simulink library "Energy_converter_Electrical_to_Mechanical"  (R2016a)
settings: Solver=ode1  StartTime=0.0  StopTime=Inf  FixedStep=0.001  RelTol=1e-3
undefined symbols (not defined in the file): API1dcac_efficiency, API2dcac_efficiency, API3dcac_efficiency, aux_power_state, AWR_InvStError, dat, DiscIntNeverNeededParam, EDCU_p_RefTqeMOT, emot_AcCmprFront_inertia, emot_AcCmprFront_nTab_3rdD, emot_AcCmprFront_pwrAC, emot_AcCmprFront_Tau, emot_AcCmprFront_trqTab_2ndD, emot_AcCmprFront_vltTab_1stD, emot_AcCmprRear_inertia, emot_AcCmprRear_nTab_3rdD, emot_AcCmprRear_pwrAC, emot_AcCmprRear_Tau, emot_AcCmprRear_trqTab_2ndD, emot_AcCmprRear_vltTab_1stD, emot_AirCmpr_inertia, emot_AirCmpr_nTab_3rdD, emot_AirCmpr_pwrAC, emot_AirCmpr_Tau, emot_AirCmpr_trqTab_2ndD, emot_AirCmpr_vltTab_1stD, emot_aircomp_power, emot_Cth_rotor, emot_Cth_stator, emot_dtrqEmotNeg, emot_dtrqEmotPtv, emot_inv_pwracTab_1st, emot_inv_pwrDC, emot_inv_pwrLoss, emot_inv_VrmsTab_2nd, emot_j, emot_mot_pwrLoss, emot_nTab_1stD, emot_pwrEtaTab_nRow, emot_pwrEtaTab_pwrTab, emot_pwrEtaTab_trqClm, emot_Rth_rotor_oil, emot_Rth_stator_oil, emot_Rth_stator_rotor, emot_tractiongroup, emot_Trotor_init, emot_trqMaxRow, emot_trqMinRow, emot_Tstator_init, emot_vltTab_3rdD, FirstDrivenAxleNoOfEmot, inv_Cth_cooling_plate, inv_Cth_diode, inv_Cth_IGBT, inv_n_IGBT_per_Switch, inv_Rth_cooling_plate_coolant, inv_Rth_PS_cooling_plate, inv_Tplate_init, inv_Tpowerstack_init, midAxleNoOfEmot ... (+6)
libraries: Electrical_converter x12, Energy_converter_Electrical_to_Mechanical x12, simulink x7
(part 4 of 8)

== system Energy_converter_Electrical_to_Mechanical/AWR_DriveEmot/EMD1_CMD_Command2 ==
  EMD1_CMD_ClearErrors : Inport
  EMD1_CMD_MotorControlMode : Inport  Port=2
  Compare To Constant : Subsystem  mask(Compare To Constant){relop===, const=1, OutDataTypeStr=boolean, ZeroCross=on}
      mask prompts: relop "Simulink:masks:Operator_MP"; const "Simulink:masks:ConstantValue_MP"; OutDataTypeStr "Simulink:masks:OutputDataType_MP"; ZeroCross "Simulink:masks:EnableZerocrossingDetection_MP"
      mask help: Simulink:masks:CompareToConstant_MD
      mask init: same as Energy_converter_Electrical_to_Mechanical/AWR_DriveEmot/EMD1_CMD_Command/Compare To Constant
      mask TypeOptions relop: == | ~= | < | <= | >= | >
      mask TypeOptions OutDataTypeStr: Simulink:masks:uint8 | Simulink:masks:boolean
      mask Callback ZeroCross: sl('zeroCrossEnable', gcbh);
      mask Display: disp(str)
  Compare To Constant1 : Subsystem  mask(Compare To Constant){relop===, const=1, OutDataTypeStr=boolean, ZeroCross=on}
      mask prompts: relop "Simulink:masks:Operator_MP"; const "Simulink:masks:ConstantValue_MP"; OutDataTypeStr "Simulink:masks:OutputDataType_MP"; ZeroCross "Simulink:masks:EnableZerocrossingDetection_MP"
      mask help: Simulink:masks:CompareToConstant_MD
      mask init: same as Energy_converter_Electrical_to_Mechanical/AWR_DriveEmot/EMD1_CMD_Command/Compare To Constant
      mask TypeOptions relop: == | ~= | < | <= | >= | >
      mask TypeOptions OutDataTypeStr: Simulink:masks:uint8 | Simulink:masks:boolean
      mask Callback ZeroCross: sl('zeroCrossEnable', gcbh);
      mask Display: disp(str)
  Constant : Constant  Value=4
  Constant3 : Constant
  Constant4 : Constant  Value=0
  Switch : Switch  Threshold=0.5
  Switch1 : Switch  Threshold=0.5
  Out_EMD1_CMD_Command : Outport
  wires:
  EMD1_CMD_MotorControlMode/1 -> Compare To Constant/1(u)
  EMD1_CMD_ClearErrors/1 -> Compare To Constant1/1(u)
  Compare To Constant1/1(y) -> Switch/2
  Switch1/1 -> Switch/3
  Constant/1 -> Switch/1
  Constant3/1 -> Switch1/1
  Constant4/1 -> Switch1/3
  Switch/1 -> Out_EMD1_CMD_Command/1
  Compare To Constant/1(y) -> Switch1/2

== system Energy_converter_Electrical_to_Mechanical/AWR_DriveEmot/EMD1_CMD_Command3 ==
  EMD1_CMD_ClearErrors : Inport
  EMD1_CMD_MotorControlMode : Inport  Port=2
  Compare To Constant : Subsystem  mask(Compare To Constant){relop===, const=1, OutDataTypeStr=boolean, ZeroCross=on}
      mask prompts: relop "Simulink:masks:Operator_MP"; const "Simulink:masks:ConstantValue_MP"; OutDataTypeStr "Simulink:masks:OutputDataType_MP"; ZeroCross "Simulink:masks:EnableZerocrossingDetection_MP"
      mask help: Simulink:masks:CompareToConstant_MD
      mask init: same as Energy_converter_Electrical_to_Mechanical/AWR_DriveEmot/EMD1_CMD_Command/Compare To Constant
      mask TypeOptions relop: == | ~= | < | <= | >= | >
      mask TypeOptions OutDataTypeStr: Simulink:masks:uint8 | Simulink:masks:boolean
      mask Callback ZeroCross: sl('zeroCrossEnable', gcbh);
      mask Display: disp(str)
  Compare To Constant1 : Subsystem  mask(Compare To Constant){relop===, const=1, OutDataTypeStr=boolean, ZeroCross=on}
      mask prompts: relop "Simulink:masks:Operator_MP"; const "Simulink:masks:ConstantValue_MP"; OutDataTypeStr "Simulink:masks:OutputDataType_MP"; ZeroCross "Simulink:masks:EnableZerocrossingDetection_MP"
      mask help: Simulink:masks:CompareToConstant_MD
      mask init: same as Energy_converter_Electrical_to_Mechanical/AWR_DriveEmot/EMD1_CMD_Command/Compare To Constant
      mask TypeOptions relop: == | ~= | < | <= | >= | >
      mask TypeOptions OutDataTypeStr: Simulink:masks:uint8 | Simulink:masks:boolean
      mask Callback ZeroCross: sl('zeroCrossEnable', gcbh);
      mask Display: disp(str)
  Constant : Constant  Value=4
  Constant3 : Constant
  Constant4 : Constant  Value=0
  Switch : Switch  Threshold=0.5
  Switch1 : Switch  Threshold=0.5
  Out_EMD1_CMD_Command : Outport
  wires:
  EMD1_CMD_MotorControlMode/1 -> Compare To Constant/1(u)
  EMD1_CMD_ClearErrors/1 -> Compare To Constant1/1(u)
  Compare To Constant1/1(y) -> Switch/2
  Switch1/1 -> Switch/3
  Constant/1 -> Switch/1
  Constant3/1 -> Switch1/1
  Constant4/1 -> Switch1/3
  Switch/1 -> Out_EMD1_CMD_Command/1
  Compare To Constant/1(y) -> Switch1/2

== system Energy_converter_Electrical_to_Mechanical/AWR_DriveEmot/Emot1_4 ==
  hvs_emot_Emot1_angVel : Inport
  voltBatHV1 : Inport  Port=2
  trqEmotDesPhy1 : Inport  Port=3
  emot_CMD1 : Inport  Port=4
  voltBatHV4 : Inport  Port=5
  trqEmotDesPhy4 : Inport  Port=6
  emot_CMD4 : Inport  Port=7
  hvs_drvEmot1Oil_Temperature : Inport  Port=8
  inv_coolant_temperature : Inport  Port=9
  Emot1_Selection : Inport  Port=10
  Emot4_Selection : Inport  Port=11
  hvs_emot_Emot4_angVel : Inport  Port=12
  hvs_drvEmot4Oil_Temperature : Inport  Port=13
  Bus Creator1 : BusCreator  Inputs=9
  Bus Creator2 : BusCreator  Inputs=9
  Bus Creator3 : BusCreator  Inputs=2
  e-Motor1 : Energy_converter_Electrical_to_Mechanical/e-Motor  SystemSampleTime=-1
  e-Motor4 : Energy_converter_Electrical_to_Mechanical/e-Motor  SystemSampleTime=-1
  emot1_4B : Outport
  wires:
  hvs_drvEmot4Oil_Temperature/1 -> e-Motor4/5
  Emot1_Selection/1 -> e-Motor1/Enable
  Emot4_Selection/1 -> e-Motor4/Enable
  Bus Creator3/1 -> emot1_4B/1  "emot1_4B"
  trqEmotDesPhy4/1 -> e-Motor4/3
  Bus Creator2/1 -> Bus Creator3/2  "emot4B"
  Bus Creator1/1 -> Bus Creator3/1  "emot1B"
  voltBatHV4/1 -> e-Motor4/2
  hvs_emot_Emot4_angVel/1 -> e-Motor4/1
  voltBatHV1/1 -> e-Motor1/2
  trqEmotDesPhy1/1 -> e-Motor1/3
  hvs_emot_Emot1_angVel/1 -> e-Motor1/1
  e-Motor1/3 -> Bus Creator1/3
  e-Motor1/4 -> Bus Creator1/4
  e-Motor1/1 -> Bus Creator1/1
  e-Motor1/2 -> Bus Creator1/2
  e-Motor1/5 -> Bus Creator1/5
  e-Motor4/1 -> Bus Creator2/1
  e-Motor4/2 -> Bus Creator2/2
  e-Motor4/3 -> Bus Creator2/3
  e-Motor4/4 -> Bus Creator2/4
  e-Motor4/5 -> Bus Creator2/5
  emot_CMD1/1 -> e-Motor1/4
  emot_CMD4/1 -> e-Motor4/4
  inv_coolant_temperature/1 -> e-Motor1/6, e-Motor4/6
  hvs_drvEmot1Oil_Temperature/1 -> e-Motor1/5
  e-Motor1/6 -> Bus Creator1/6
  e-Motor1/7 -> Bus Creator1/7
  e-Motor1/9 -> Bus Creator1/9
  e-Motor1/8 -> Bus Creator1/8
  e-Motor4/6 -> Bus Creator2/6
  e-Motor4/7 -> Bus Creator2/7
  e-Motor4/8 -> Bus Creator2/8
  e-Motor4/9 -> Bus Creator2/9

== system Energy_converter_Electrical_to_Mechanical/AWR_DriveEmot/Emot2_3 ==
  hvs_emot_Emot2_angVel : Inport
  voltBatHV2 : Inport  Port=2
  trqEmotDesPhy2 : Inport  Port=3
  emot_CMD2 : Inport  Port=4
  voltBatHV3 : Inport  Port=5
  trqEmotDesPhy3 : Inport  Port=6
  emot_CMD3 : Inport  Port=7
  hvs_drvEmot2Oil_Temperature : Inport  Port=8
  inv_coolant_temperature : Inport  Port=9
  Emot2_Selection : Inport  Port=10
  Emot3_Selection : Inport  Port=11
  hvs_emot_Emot3_angVel : Inport  Port=12
  hvs_drvEmot3Oil_Temperature : Inport  Port=13
  Bus Creator1 : BusCreator  Inputs=9
  Bus Creator2 : BusCreator  Inputs=9
  Bus Creator3 : BusCreator  Inputs=2
  e-Motor2 : Energy_converter_Electrical_to_Mechanical/e-Motor  SystemSampleTime=-1
  e-Motor3 : Energy_converter_Electrical_to_Mechanical/e-Motor  SystemSampleTime=-1
  emot2_3B : Outport
  wires:
  hvs_drvEmot3Oil_Temperature/1 -> e-Motor3/5
  Emot3_Selection/1 -> e-Motor3/Enable
  Emot2_Selection/1 -> e-Motor2/Enable
  emot_CMD3/1 -> e-Motor3/4
  emot_CMD2/1 -> e-Motor2/4
  e-Motor3/5 -> Bus Creator2/5
  e-Motor3/4 -> Bus Creator2/4
  e-Motor3/3 -> Bus Creator2/3
  e-Motor3/2 -> Bus Creator2/2
  e-Motor3/1 -> Bus Creator2/1
  e-Motor2/5 -> Bus Creator1/5
  e-Motor2/2 -> Bus Creator1/2
  e-Motor2/1 -> Bus Creator1/1
  e-Motor2/4 -> Bus Creator1/4
  e-Motor2/3 -> Bus Creator1/3
  hvs_emot_Emot2_angVel/1 -> e-Motor2/1
  trqEmotDesPhy2/1 -> e-Motor2/3
  voltBatHV2/1 -> e-Motor2/2
  hvs_emot_Emot3_angVel/1 -> e-Motor3/1
  voltBatHV3/1 -> e-Motor3/2
  Bus Creator1/1 -> Bus Creator3/1  "emot2B"
  Bus Creator2/1 -> Bus Creator3/2  "emot3B"
  trqEmotDesPhy3/1 -> e-Motor3/3
  Bus Creator3/1 -> emot2_3B/1  "emot2_3B"
  hvs_drvEmot2Oil_Temperature/1 -> e-Motor2/5
  inv_coolant_temperature/1 -> e-Motor2/6, e-Motor3/6
  e-Motor3/7 -> Bus Creator2/7
  e-Motor3/6 -> Bus Creator2/6
  e-Motor3/8 -> Bus Creator2/8
  e-Motor3/9 -> Bus Creator2/9
  e-Motor2/6 -> Bus Creator1/6
  e-Motor2/7 -> Bus Creator1/7
  e-Motor2/9 -> Bus Creator1/9
  e-Motor2/8 -> Bus Creator1/8

== system Energy_converter_Electrical_to_Mechanical/AWR_DriveEmot/MotorSelection ==
  MidAxle : Constant  Value=FirstDrivenAxleNoOfEmot
  RearAxle : Constant  Value=SecondDrivenAxleNoOfEmot
  Truth Table : Truth Table  TreatAsAtomicUnit=on
  Emot1_Selection : Outport
  Emot2_Selection : Outport  Port=2
  Emot3_Selection : Outport  Port=3
  Emot4_Selection : Outport  Port=4
  wires:
  Truth Table/4(y4) -> Emot4_Selection/1
  Truth Table/3(y3) -> Emot3_Selection/1
  Truth Table/2(y2) -> Emot2_Selection/1
  Truth Table/1(y1) -> Emot1_Selection/1
  RearAxle/1 -> Truth Table/2(u2)
  MidAxle/1 -> Truth Table/1(u1)

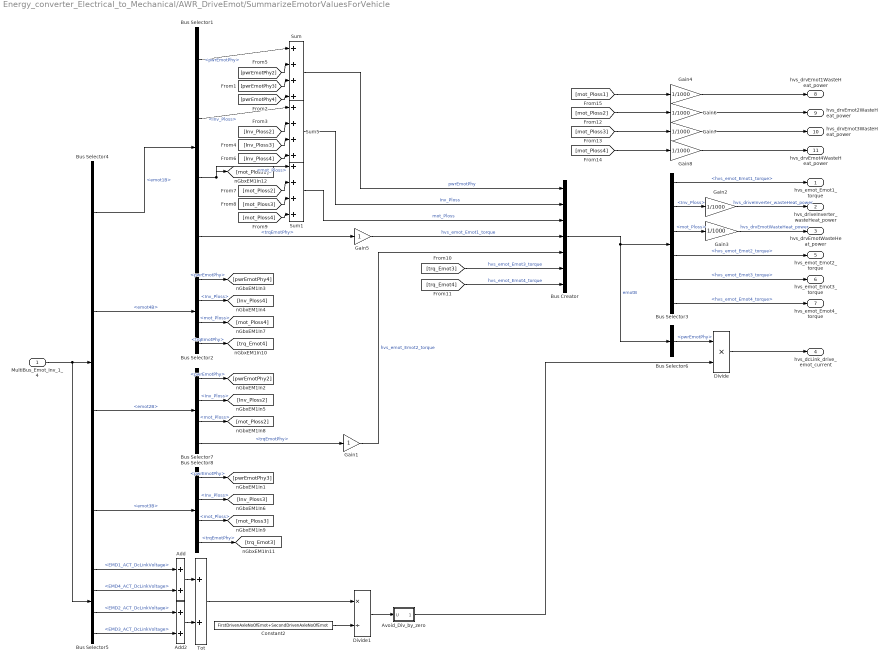
== system Energy_converter_Electrical_to_Mechanical/AWR_DriveEmot/SummarizeEmotorValuesForVehicle ==
  MultiBus_Emot_Inv_1_4 : Inport
  Add : Sum
  Add2 : Sum
  Avoid_Div_by_zero : Subsystem
  Bus Creator : BusCreator  Inputs=7
  Bus Selector{1..2,7..8} (4 alike) : BusSelector  OutputSignals=pwrEmotPhy,Inv_Ploss,mot_Ploss,trqEmotPhy
  Bus Selector3 : BusSelector  OutputSignals=hvs_emot_Emot1_torque,Inv_Ploss,mot_Ploss,hvs_emot_Emot2_torque,hvs_emot_Emot3_torque,hvs_emot_Emot4_torque
  Bus Selector4 : BusSelector  OutputSignals=emot1_4B.emot1B,emot1_4B.emot4B,emot2_3B.emot2B,emot2_3B.emot3B
  Bus Selector5 : BusSelector  OutputSignals=awr1_4B.awr1B.EMD1_ACT_DcLinkVoltage,awr1_4B.awr4B.EMD4_ACT_DcLinkVoltage,awr2_3B.awr2B.EMD2_ACT_DcLinkVoltage,awr2_3B.awr3B.EMD3_ACT_DcLinkVoltage
  Bus Selector6 : BusSelector  OutputSignals=pwrEmotPhy
  Constant2 : Constant  Value=FirstDrivenAxleNoOfEmot+SecondDrivenAxleNoOfEmot
  Divide : Product  Inputs=**
  Divide1 : Product  Inputs=*/
  Gain1 : Gain
  Gain{2..4,6..8} (6 alike) : Gain  Gain=1/1000
  Gain5 : Gain
  Sum : Sum  Inputs=|++++
  Sum1 : Sum  Inputs=|++++
  Sum5 : Sum  Inputs=|++++
  Tot : Sum
  hvs_emot_Emot1_torque : Outport
  hvs_driveInverter_wasteHeat_power : Outport  Port=2
  hvs_drvEmotWasteHeat_power : Outport  Port=3
  hvs_dcLink_drive_emot_current : Outport  Port=4
  hvs_emot_Emot2_torque : Outport  Port=5
  hvs_emot_Emot3_torque : Outport  Port=6
  hvs_emot_Emot4_torque : Outport  Port=7
  hvs_drvEmot1WasteHeat_power : Outport  Port=8
  hvs_drvEmot2WasteHeat_power : Outport  Port=9
  hvs_drvEmot3WasteHeat_power : Outport  Port=10
  hvs_drvEmot4WasteHeat_power : Outport  Port=11
  wires:
  Gain8/1 -> hvs_drvEmot4WasteHeat_power/1
  Gain7/1 -> hvs_drvEmot3WasteHeat_power/1
  Gain6/1 -> hvs_drvEmot2WasteHeat_power/1
  Gain4/1 -> hvs_drvEmot1WasteHeat_power/1
  [mot_Ploss4] -> Gain8/1
  [mot_Ploss3] -> Gain7/1
  [mot_Ploss2] -> Gain6/1
  [mot_Ploss1] -> Gain4/1
  Bus Selector3/6 -> hvs_emot_Emot4_torque/1  "<hvs_emot_Emot4_torque>"
  Bus Selector3/5 -> hvs_emot_Emot3_torque/1  "<hvs_emot_Emot3_torque>"
  Bus Selector3/4 -> hvs_emot_Emot2_torque/1  "<hvs_emot_Emot2_torque>"
  Bus Selector3/1 -> hvs_emot_Emot1_torque/1  "<hvs_emot_Emot1_torque>"
  [trq_Emot4] -> Bus Creator/7  "hvs_emot_Emot4_torque"
  [trq_Emot3] -> Bus Creator/6  "hvs_emot_Emot3_torque"
  Bus Selector2/4 -> [trq_Emot4]  "<trqEmotPhy>"
  Tot/1 -> Divide1/1
  Constant2/1 -> Divide1/2
  Add2/1 -> Tot/2
  Bus Selector5/4 -> Add2/2  "<EMD3_ACT_DcLinkVoltage>"
  Bus Selector5/3 -> Add2/1  "<EMD2_ACT_DcLinkVoltage>"
  Gain1/1 -> Bus Creator/5  "hvs_emot_Emot2_torque"
  Bus Selector8/4 -> [trq_Emot3]  "<trqEmotPhy>"
  Bus Selector7/4 -> Gain1/1  "<trqEmotPhy>"
  [mot_Ploss4] -> Sum1/4
  [mot_Ploss3] -> Sum1/3
  [mot_Ploss2] -> Sum1/2
  Bus Selector8/3 -> [mot_Ploss3]  "<mot_Ploss>"
  Bus Selector7/3 -> [mot_Ploss2]  "<mot_Ploss>"
  Bus Selector8/2 -> [Inv_Ploss3]  "<Inv_Ploss>"
  Bus Selector7/2 -> [Inv_Ploss2]  "<Inv_Ploss>"
  [Inv_Ploss4] -> Sum5/4
  [Inv_Ploss3] -> Sum5/3
  [Inv_Ploss2] -> Sum5/2
  [pwrEmotPhy4] -> Sum/4
  [pwrEmotPhy3] -> Sum/3
  [pwrEmotPhy2] -> Sum/2
  Bus Selector2/1 -> [pwrEmotPhy4]  "<pwrEmotPhy>"
  Bus Selector8/1 -> [pwrEmotPhy3]  "<pwrEmotPhy>"
  Bus Selector7/1 -> [pwrEmotPhy2]  "<pwrEmotPhy>"
  Bus Selector4/3 -> Bus Selector7/1  "<emot2B>"
  Bus Selector4/4 -> Bus Selector8/1  "<emot3B>"
  Gain3/1 -> hvs_drvEmotWasteHeat_power/1  "hvs_drvEmotWasteHeat_power"
  Bus Selector3/3 -> Gain3/1  "<mot_Ploss>"
  Gain2/1 -> hvs_driveInverter_wasteHeat_power/1  "hvs_driveInverter_wasteHeat_power"
  Bus Selector3/2 -> Gain2/1  "<Inv_Ploss>"
  Divide/1 -> hvs_dcLink_drive_emot_current/1
  Avoid_Div_by_zero/1(1/U) -> Divide/2
  Bus Selector6/1 -> Divide/1  "<pwrEmotPhy>"
  Divide1/1 -> Avoid_Div_by_zero/1(U)
  Add/1 -> Tot/1
  Bus Selector5/2 -> Add/2  "<EMD4_ACT_DcLinkVoltage>"
  Bus Selector5/1 -> Add/1  "<EMD1_ACT_DcLinkVoltage>"
  Bus Creator/1 -> Bus Selector6/1, Bus Selector3/1  "emotB"
  MultiBus_Emot_Inv_1_4/1 -> Bus Selector4/1, Bus Selector5/1
  Bus Selector4/1 -> Bus Selector1/1  "<emot1B>"
  Bus Selector4/2 -> Bus Selector2/1  "<emot4B>"
  Bus Selector1/1 -> Sum/1  "<pwrEmotPhy>"
  Bus Selector1/2 -> Sum5/1  "<Inv_Ploss>"
  Bus Selector2/2 -> [Inv_Ploss4]  "<Inv_Ploss>"
  Bus Selector1/3 -> Sum1/1, [mot_Ploss1]  "<mot_Ploss>"
  Bus Selector2/3 -> [mot_Ploss4]  "<mot_Ploss>"
  Bus Selector1/4 -> Gain5/1  "<trqEmotPhy>"
  Sum/1 -> Bus Creator/1  "pwrEmotPhy"
  Sum5/1 -> Bus Creator/2  "Inv_Ploss"
  Sum1/1 -> Bus Creator/3  "mot_Ploss"
  Gain5/1 -> Bus Creator/4  "hvs_emot_Emot1_torque"

== system Energy_converter_Electrical_to_Mechanical/AWR_DriveEmot/percent_to_Nm ==
  Percentage_Torque : Inport
  Reference_Torque : Inport  Port=2
  Constant : Constant  Value=100
  Divide : Product  Inputs=*/
  Product : Product  RndMeth=Zero
  Torque_Nm : Outport
  wires:
  Percentage_Torque/1 -> Product/1  "Percentage_Torque"
  Divide/1 -> Torque_Nm/1  "Torque_Nm"
  Reference_Torque/1 -> Product/2  "Reference_Torque"
  Product/1 -> Divide/1
  Constant/1 -> Divide/2

== system Energy_converter_Electrical_to_Mechanical/AWR_DriveEmot/percent_to_Nm1 ==
  Percentage_Torque : Inport
  Reference_Torque : Inport  Port=2
  Constant : Constant  Value=100
  Divide : Product  Inputs=*/
  Product : Product  RndMeth=Zero
  Torque_Nm : Outport
  wires:
  Percentage_Torque/1 -> Product/1  "Percentage_Torque"
  Divide/1 -> Torque_Nm/1  "Torque_Nm"
  Reference_Torque/1 -> Product/2  "Reference_Torque"
  Product/1 -> Divide/1
  Constant/1 -> Divide/2

== system Energy_converter_Electrical_to_Mechanical/AWR_DriveEmot/percent_to_Nm2 ==
  Percentage_Torque : Inport
  Reference_Torque : Inport  Port=2
  Constant : Constant  Value=100
  Divide : Product  Inputs=*/
  Product : Product  RndMeth=Zero
  Torque_Nm : Outport
  wires:
  Percentage_Torque/1 -> Product/1  "Percentage_Torque"
  Divide/1 -> Torque_Nm/1  "Torque_Nm"
  Reference_Torque/1 -> Product/2  "Reference_Torque"
  Product/1 -> Divide/1
  Constant/1 -> Divide/2

== system Energy_converter_Electrical_to_Mechanical/AWR_DriveEmot/percent_to_Nm3 ==
  Percentage_Torque : Inport
  Reference_Torque : Inport  Port=2
  Constant : Constant  Value=100
  Divide : Product  Inputs=*/
  Product : Product  RndMeth=Zero
  Torque_Nm : Outport
  wires:
  Percentage_Torque/1 -> Product/1  "Percentage_Torque"
  Divide/1 -> Torque_Nm/1  "Torque_Nm"
  Reference_Torque/1 -> Product/2  "Reference_Torque"
  Product/1 -> Divide/1
  Constant/1 -> Divide/2

== system Energy_converter_Electrical_to_Mechanical/AWR_DriveEmot_Gen2/AWR 1 TX ==
  IN_EMD1_ACT_DcLinkVoltage : Inport
  IN_EMD1_ACT_DigitalInput1 : Inport  Port=2
  IN_EMD1_ACT_MaximumAvailableTorque : Inport  Port=3
  IN_EMD1_ACT_DcLinkPower : Inport  Port=4
  IN_EMD1_ACT_MotorSpeed : Inport  Port=5
  IN_EMD1_ACT_Torque : Inport  Port=6
  IN_EMD1_ACT_InverterState : Inport  Port=7
  IN_EMD1_ACT_ReferenceTorqueLimited : Inport  Port=8
  IN_EMD1_ACT_MaxJunctionTemperature : Inport  Port=9
  IN_EMD1_ACT_MotorTemperature : Inport  Port=10
  IN_EMD1_ACT_InverterLosses : Inport  Port=11
  IN_EMD1_ACT_MotorLosses : Inport  Port=12
  Constant3 : Constant  Value=RefTqeMOT
  Constant39 : Constant  Value=RefTqeMOT
  Constant5 : Constant  Value=RefTqeMOT
  Nm_to_percent : Subsystem
  Nm_to_percent1 : Subsystem
  Nm_to_percent2 : Subsystem
  hvs_EMD1_ACT_DigitalInput1 : Outport
  hvs_EMD1_ACT_InverterState : Outport  Port=2
  hvs_EMD1_ACT_MaxAvailableTorque : Outport  Port=3
  hvs_EMD1_ACT_ReferenceTorqueLim : Outport  Port=4
  hvs_EMD1_ACT_Torque : Outport  Port=5
  hvs_EMD1_ACT_DcLinkPower : Outport  Port=6
  hvs_EMD1_ACT_MotorSpeed : Outport  Port=7
  hvs_EMD1_ACT_DcLinkVoltage : Outport  Port=8
  hvs_EMD1_ACT_MaxJunctionTemp : Outport  Port=9
  hvs_EMD1_ACT_MotorTemperature : Outport  Port=10
  hvs_EMD1_ACT_InverterLosses : Outport  Port=11
  hvs_EMD1_ACT_MotorLosses : Outport  Port=12
  wires:
  Constant5/1 -> Nm_to_percent1/2(Reference_Torque)
  IN_EMD1_ACT_ReferenceTorqueLimited/1 -> Nm_to_percent1/1(Nm_Torque)  "EMD1_ACT_ReferenceTorqueLimited"
  IN_EMD1_ACT_InverterState/1 -> hvs_EMD1_ACT_InverterState/1  "hvs_EMD1_ACT_InverterState"
  IN_EMD1_ACT_DcLinkPower/1 -> hvs_EMD1_ACT_DcLinkPower/1  "hvs_EMD1_ACT_DcLinkPower"
  IN_EMD1_ACT_DcLinkVoltage/1 -> hvs_EMD1_ACT_DcLinkVoltage/1  "hvs_EMD1_ACT_DcLinkVoltage"
  Nm_to_percent/1(Torque_Percentage) -> hvs_EMD1_ACT_MaxAvailableTorque/1  "hvs_EMD1_ACT_MaxAvailableTorque"
  Nm_to_percent1/1(Torque_Percentage) -> hvs_EMD1_ACT_ReferenceTorqueLim/1  "hvs_EMD1_ACT_ReferenceTorqueLim"
  IN_EMD1_ACT_MotorSpeed/1 -> hvs_EMD1_ACT_MotorSpeed/1  "hvs_EMD1_ACT_MotorSpeed"
  IN_EMD1_ACT_Torque/1 -> Nm_to_percent2/1(Nm_Torque)
  IN_EMD1_ACT_MaxJunctionTemperature/1 -> hvs_EMD1_ACT_MaxJunctionTemp/1  "hvs_EMD1_ACT_MaxJunctionTemp"
  IN_EMD1_ACT_MotorTemperature/1 -> hvs_EMD1_ACT_MotorTemperature/1  "hvs_EMD1_ACT_MotorTemperature"
  IN_EMD1_ACT_DigitalInput1/1 -> hvs_EMD1_ACT_DigitalInput1/1  "hvs_EMD1_ACT_DigitalInput1"
  IN_EMD1_ACT_MaximumAvailableTorque/1 -> Nm_to_percent/1(Nm_Torque)  "EMD1_ACT_MaximumAvailableTorque"
  Constant3/1 -> Nm_to_percent/2(Reference_Torque)
  Nm_to_percent2/1(Torque_Percentage) -> hvs_EMD1_ACT_Torque/1  "hvs_EMD1_ACT_Torque"
  Constant39/1 -> Nm_to_percent2/2(Reference_Torque)
  IN_EMD1_ACT_InverterLosses/1 -> hvs_EMD1_ACT_InverterLosses/1  "hvs_EMD1_ACT_InverterLosses"
  IN_EMD1_ACT_MotorLosses/1 -> hvs_EMD1_ACT_MotorLosses/1  "hvs_EMD1_ACT_MotorLosses"

== system Energy_converter_Electrical_to_Mechanical/AWR_DriveEmot_Gen2/AWR 2 TX ==
  IN_EMD2_ACT_DcLinkVoltage : Inport
  IN_EMD2_ACT_DigitalInput1 : Inport  Port=2
  IN_EMD2_ACT_MaximumAvailableTorque : Inport  Port=3
  IN_EMD2_ACT_DcLinkPower : Inport  Port=4
  IN_EMD2_ACT_MotorSpeed : Inport  Port=5
  IN_EMD2_ACT_Torque : Inport  Port=6
  IN_EMD2_ACT_InverterState : Inport  Port=7
  IN_EMD2_ACT_ReferenceTorqueLimited : Inport  Port=8
  IN_EMD2_ACT_MaxJunctionTemperature : Inport  Port=9
  IN_EMD2_ACT_MotorTemperature : Inport  Port=10
  IN_EMD2_ACT_InverterLosses : Inport  Port=11
  IN_EMD2_ACT_MotorLosses : Inport  Port=12
  Constant3 : Constant  Value=RefTqeMOT
  Constant39 : Constant  Value=RefTqeMOT
  Constant5 : Constant  Value=RefTqeMOT
  Nm_to_percent : Subsystem
  Nm_to_percent1 : Subsystem
  Nm_to_percent2 : Subsystem
  hvs_EMD2_ACT_DigitalInput1 : Outport
  hvs_EMD2_ACT_InverterState : Outport  Port=2
  hvs_EMD2_ACT_MaxAvailableTorque : Outport  Port=3
  hvs_EMD2_ACT_ReferenceTorqueLim : Outport  Port=4
  hvs_EMD2_ACT_Torque : Outport  Port=5
  hvs_EMD2_ACT_DcLinkPower : Outport  Port=6
  hvs_EMD2_ACT_MotorSpeed : Outport  Port=7
  hvs_EMD2_ACT_DcLinkVoltage : Outport  Port=8
  hvs_EMD2_ACT_MaxJunctionTemp : Outport  Port=9
  hvs_EMD2_ACT_MotorTemperature : Outport  Port=10
  hvs_EMD2_ACT_InverterLosses : Outport  Port=11
  hvs_EMD2_ACT_MotorLosses : Outport  Port=12
  wires:
  Constant5/1 -> Nm_to_percent1/2(Reference_Torque)
  IN_EMD2_ACT_ReferenceTorqueLimited/1 -> Nm_to_percent1/1(Nm_Torque)  "EMD1_ACT_ReferenceTorqueLimited"
  IN_EMD2_ACT_InverterState/1 -> hvs_EMD2_ACT_InverterState/1  "hvs_EMD2_ACT_InverterState"
  IN_EMD2_ACT_DcLinkPower/1 -> hvs_EMD2_ACT_DcLinkPower/1  "hvs_EMD2_ACT_DcLinkPower"
  IN_EMD2_ACT_DcLinkVoltage/1 -> hvs_EMD2_ACT_DcLinkVoltage/1  "hvs_EMD2_ACT_DcLinkVoltage"
  Nm_to_percent/1(Torque_Percentage) -> hvs_EMD2_ACT_MaxAvailableTorque/1  "hvs_EMD2_ACT_MaxAvailableTorque"
  Nm_to_percent1/1(Torque_Percentage) -> hvs_EMD2_ACT_ReferenceTorqueLim/1  "hvs_EMD2_ACT_ReferenceTorqueLim"
  IN_EMD2_ACT_MotorSpeed/1 -> hvs_EMD2_ACT_MotorSpeed/1  "hvs_EMD2_ACT_MotorSpeed"
  IN_EMD2_ACT_Torque/1 -> Nm_to_percent2/1(Nm_Torque)
  IN_EMD2_ACT_MaxJunctionTemperature/1 -> hvs_EMD2_ACT_MaxJunctionTemp/1  "hvs_EMD2_ACT_MaxJunctionTemp"
  IN_EMD2_ACT_MotorTemperature/1 -> hvs_EMD2_ACT_MotorTemperature/1  "hvs_EMD2_ACT_MotorTemperature"
  IN_EMD2_ACT_DigitalInput1/1 -> hvs_EMD2_ACT_DigitalInput1/1  "hvs_EMD2_ACT_DigitalInput1"
  IN_EMD2_ACT_MaximumAvailableTorque/1 -> Nm_to_percent/1(Nm_Torque)  "EMD1_ACT_MaximumAvailableTorque"
  Constant3/1 -> Nm_to_percent/2(Reference_Torque)
  Nm_to_percent2/1(Torque_Percentage) -> hvs_EMD2_ACT_Torque/1  "hvs_EMD2_ACT_Torque"
  Constant39/1 -> Nm_to_percent2/2(Reference_Torque)
  IN_EMD2_ACT_InverterLosses/1 -> hvs_EMD2_ACT_InverterLosses/1  "hvs_EMD2_ACT_InverterLosses"
  IN_EMD2_ACT_MotorLosses/1 -> hvs_EMD2_ACT_MotorLosses/1  "hvs_EMD2_ACT_MotorLosses"

== system Energy_converter_Electrical_to_Mechanical/AWR_DriveEmot_Gen2/AWR 3 TX ==
  IN_EMD3_ACT_DcLinkVoltage : Inport
  IN_EMD3_ACT_DigitalInput1 : Inport  Port=2
  IN_EMD3_ACT_MaximumAvailableTorque : Inport  Port=3
  IN_EMD3_ACT_DcLinkPower : Inport  Port=4
  IN_EMD3_ACT_MotorSpeed : Inport  Port=5
  IN_EMD3_ACT_Torque : Inport  Port=6
  IN_EMD3_ACT_InverterState : Inport  Port=7
  IN_EMD3_ACT_ReferenceTorqueLimited : Inport  Port=8
  IN_EMD3_ACT_MaxJunctionTemperature : Inport  Port=9
  IN_EMD3_ACT_MotorTemperature : Inport  Port=10
  IN_EMD3_ACT_InverterLosses : Inport  Port=11
  IN_EMD3_ACT_MotorLosses : Inport  Port=12
  Constant3 : Constant  Value=RefTqeMOT
  Constant39 : Constant  Value=RefTqeMOT
  Constant5 : Constant  Value=RefTqeMOT
  Nm_to_percent : Subsystem
  Nm_to_percent1 : Subsystem
  Nm_to_percent2 : Subsystem
  hvs_EMD3_ACT_DigitalInput1 : Outport
  hvs_EMD3_ACT_InverterState : Outport  Port=2
  hvs_EMD3_ACT_MaxAvailableTorque : Outport  Port=3
  hvs_EMD3_ACT_ReferenceTorqueLim : Outport  Port=4
  hvs_EMD3_ACT_Torque : Outport  Port=5
  hvs_EMD3_ACT_DcLinkPower : Outport  Port=6
  hvs_EMD3_ACT_MotorSpeed : Outport  Port=7
  hvs_EMD3_ACT_DcLinkVoltage : Outport  Port=8
  hvs_EMD3_ACT_MaxJunctionTemp : Outport  Port=9
  hvs_EMD3_ACT_MotorTemperature : Outport  Port=10
  hvs_EMD3_ACT_InverterLosses : Outport  Port=11
  hvs_EMD3_ACT_MotorLosses : Outport  Port=12
  wires:
  Constant39/1 -> Nm_to_percent2/2(Reference_Torque)
  Nm_to_percent2/1(Torque_Percentage) -> hvs_EMD3_ACT_Torque/1  "hvs_EMD3_ACT_Torque"
  Constant3/1 -> Nm_to_percent/2(Reference_Torque)
  IN_EMD3_ACT_MaximumAvailableTorque/1 -> Nm_to_percent/1(Nm_Torque)  "EMD1_ACT_MaximumAvailableTorque"
  IN_EMD3_ACT_DigitalInput1/1 -> hvs_EMD3_ACT_DigitalInput1/1  "hvs_EMD3_ACT_DigitalInput1"
  IN_EMD3_ACT_MotorTemperature/1 -> hvs_EMD3_ACT_MotorTemperature/1  "hvs_EMD3_ACT_MotorTemperature"
  IN_EMD3_ACT_MaxJunctionTemperature/1 -> hvs_EMD3_ACT_MaxJunctionTemp/1  "hvs_EMD3_ACT_MaxJunctionTemp"
  IN_EMD3_ACT_Torque/1 -> Nm_to_percent2/1(Nm_Torque)
  IN_EMD3_ACT_MotorSpeed/1 -> hvs_EMD3_ACT_MotorSpeed/1  "hvs_EMD3_ACT_MotorSpeed"
  Nm_to_percent1/1(Torque_Percentage) -> hvs_EMD3_ACT_ReferenceTorqueLim/1  "hvs_EMD3_ACT_ReferenceTorqueLim"
  Nm_to_percent/1(Torque_Percentage) -> hvs_EMD3_ACT_MaxAvailableTorque/1  "hvs_EMD3_ACT_MaxAvailableTorque"
  IN_EMD3_ACT_DcLinkVoltage/1 -> hvs_EMD3_ACT_DcLinkVoltage/1  "hvs_EMD3_ACT_DcLinkVoltage"
  IN_EMD3_ACT_DcLinkPower/1 -> hvs_EMD3_ACT_DcLinkPower/1  "hvs_EMD3_ACT_DcLinkPower"
  IN_EMD3_ACT_InverterState/1 -> hvs_EMD3_ACT_InverterState/1  "hvs_EMD3_ACT_InverterState"
  IN_EMD3_ACT_ReferenceTorqueLimited/1 -> Nm_to_percent1/1(Nm_Torque)  "EMD1_ACT_ReferenceTorqueLimited"
  Constant5/1 -> Nm_to_percent1/2(Reference_Torque)
  IN_EMD3_ACT_InverterLosses/1 -> hvs_EMD3_ACT_InverterLosses/1  "hvs_EMD3_ACT_InverterLosses"
  IN_EMD3_ACT_MotorLosses/1 -> hvs_EMD3_ACT_MotorLosses/1  "hvs_EMD3_ACT_MotorLosses"

== system Energy_converter_Electrical_to_Mechanical/AWR_DriveEmot_Gen2/AWR 4 TX ==
  IN_EMD4_ACT_DcLinkVoltage : Inport
  IN_EMD4_ACT_DigitalInput1 : Inport  Port=2
  IN_EMD4_ACT_MaximumAvailableTorque : Inport  Port=3
  IN_EMD4_ACT_DcLinkPower : Inport  Port=4
  IN_EMD4_ACT_MotorSpeed : Inport  Port=5
  IN_EMD4_ACT_Torque : Inport  Port=6
  IN_EMD4_ACT_InverterState : Inport  Port=7
  IN_EMD4_ACT_ReferenceTorqueLimited : Inport  Port=8
  IN_EMD4_ACT_MaxJunctionTemperature : Inport  Port=9
  IN_EMD4_ACT_MotorTemperature : Inport  Port=10
  IN_EMD4_ACT_InverterLosses : Inport  Port=11
  IN_EMD4_ACT_MotorLosses : Inport  Port=12
  Constant3 : Constant  Value=RefTqeMOT
  Constant39 : Constant  Value=RefTqeMOT
  Constant5 : Constant  Value=RefTqeMOT
  Nm_to_percent : Subsystem
  Nm_to_percent1 : Subsystem
  Nm_to_percent2 : Subsystem
  hvs_EMD4_ACT_DigitalInput1 : Outport
  hvs_EMD4_ACT_InverterState : Outport  Port=2
  hvs_EMD4_ACT_MaxAvailableTorque : Outport  Port=3
  hvs_EMD4_ACT_ReferenceTorqueLim : Outport  Port=4
  hvs_EMD4_ACT_Torque : Outport  Port=5
  hvs_EMD4_ACT_DcLinkPower : Outport  Port=6
  hvs_EMD4_ACT_MotorSpeed : Outport  Port=7
  hvs_EMD4_ACT_DcLinkVoltage : Outport  Port=8
  hvs_EMD4_ACT_MaxJunctionTemperature : Outport  Port=9
  hvs_EMD4_ACT_MotorTemperature : Outport  Port=10
  hvs_EMD4_ACT_InverterLosses : Outport  Port=11
  hvs_EMD4_ACT_MotorLosses : Outport  Port=12
  wires:
  Constant5/1 -> Nm_to_percent1/2(Reference_Torque)
  IN_EMD4_ACT_ReferenceTorqueLimited/1 -> Nm_to_percent1/1(Nm_Torque)  "EMD4_ACT_ReferenceTorqueLimited"
  IN_EMD4_ACT_InverterState/1 -> hvs_EMD4_ACT_InverterState/1  "hvs_EMD4_ACT_InverterState"
  IN_EMD4_ACT_DcLinkPower/1 -> hvs_EMD4_ACT_DcLinkPower/1  "hvs_EMD4_ACT_DcLinkPower"
  IN_EMD4_ACT_DcLinkVoltage/1 -> hvs_EMD4_ACT_DcLinkVoltage/1  "hvs_EMD4_ACT_DcLinkVoltage"
  Nm_to_percent/1(Torque_Percentage) -> hvs_EMD4_ACT_MaxAvailableTorque/1  "hvs_EMD4_ACT_MaxAvailableTorque"
  IN_EMD4_ACT_MotorSpeed/1 -> hvs_EMD4_ACT_MotorSpeed/1  "hvs_EMD4_ACT_MotorSpeed"
  IN_EMD4_ACT_Torque/1 -> Nm_to_percent2/1(Nm_Torque)
  IN_EMD4_ACT_MaxJunctionTemperature/1 -> hvs_EMD4_ACT_MaxJunctionTemperature/1  "hvs_EMD4_ACT_MaxJunctionTemperature"
  IN_EMD4_ACT_MotorTemperature/1 -> hvs_EMD4_ACT_MotorTemperature/1  "hvs_EMD4_ACT_MotorTemperature"
  Nm_to_percent1/1(Torque_Percentage) -> hvs_EMD4_ACT_ReferenceTorqueLim/1  "hvs_EMD4_ACT_ReferenceTorqueLim"
  IN_EMD4_ACT_DigitalInput1/1 -> hvs_EMD4_ACT_DigitalInput1/1  "hvs_EMD4_ACT_DigitalInput1"
  IN_EMD4_ACT_MaximumAvailableTorque/1 -> Nm_to_percent/1(Nm_Torque)  "EMD2_ACT_MaximumAvailableTorque"
  Constant3/1 -> Nm_to_percent/2(Reference_Torque)
  Constant39/1 -> Nm_to_percent2/2(Reference_Torque)
  Nm_to_percent2/1(Torque_Percentage) -> hvs_EMD4_ACT_Torque/1  "hvs_EMD4_ACT_Torque"
  IN_EMD4_ACT_InverterLosses/1 -> hvs_EMD4_ACT_InverterLosses/1  "hvs_EMD4_ACT_InverterLosses"
  IN_EMD4_ACT_MotorLosses/1 -> hvs_EMD4_ACT_MotorLosses/1  "hvs_EMD4_ACT_MotorLosses"

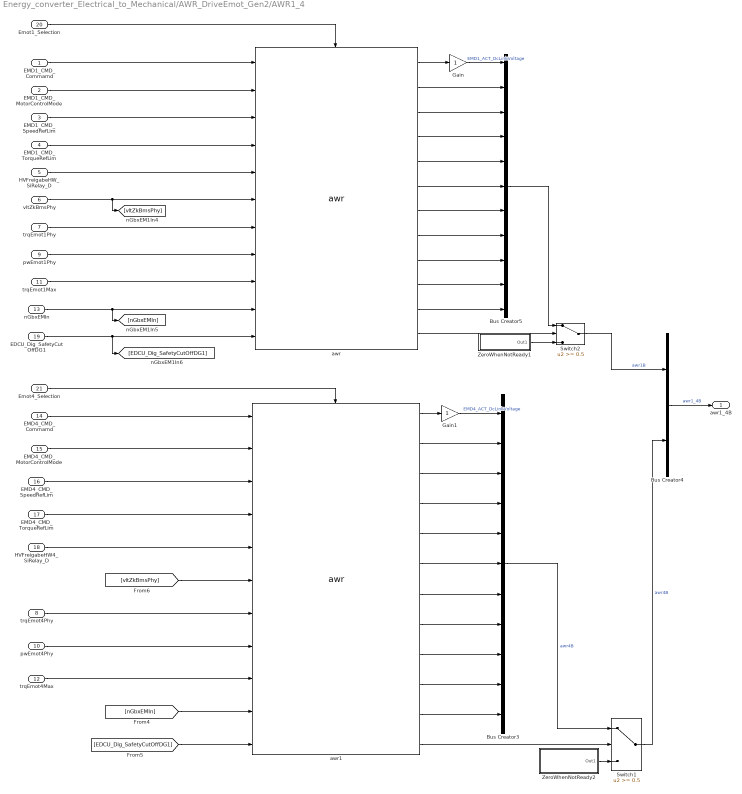
== system Energy_converter_Electrical_to_Mechanical/AWR_DriveEmot_Gen2/AWR1_4 ==
  EMD1_CMD_Commamd : Inport
  EMD1_CMD_MotorControlMode : Inport  Port=2
  EMD1_CMD_SpeedRefLim : Inport  Port=3
  EMD1_CMD_TorqueRefLim : Inport  Port=4
  HVFreigabeHW_SiRelay_D : Inport  Port=5
  vltZkBmsPhy : Inport  Port=6
  trqEmot1Phy : Inport  Port=7
  trqEmot4Phy : Inport  Port=8
  pwEmot1Phy : Inport  Port=9
  pwEmot4Phy : Inport  Port=10
  trqEmot1Max : Inport  Port=11
  trqEmot4Max : Inport  Port=12
  nGbxEMIn : Inport  Port=13
  EMD4_CMD_Commamd : Inport  Port=14
  EMD4_CMD_MotorControlMode : Inport  Port=15
  EMD4_CMD_SpeedRefLim : Inport  Port=16
  EMD4_CMD_TorqueRefLim : Inport  Port=17
  HVFreigabeHW4_SiRelay_D : Inport  Port=18
  EDCU_Dig_SafetyCutOffDG1 : Inport  Port=19
  Emot1_Selection : Inport  Port=20
  Emot4_Selection : Inport  Port=21
  Bus Creator3 : BusCreator  Inputs=11
  Bus Creator4 : BusCreator  Inputs=2
  Bus Creator5 : BusCreator  Inputs=11
  Gain : Gain
  Gain1 : Gain
  Switch1 : Switch  Threshold=0.5
  Switch2 : Switch  Threshold=0.5
  ZeroWhenNotReady1 : Subsystem  TreatAsAtomicUnit=on
  ZeroWhenNotReady2 : Subsystem  TreatAsAtomicUnit=on
  awr : Electrical_converter/awr  SystemSampleTime=-1
  awr1 : Electrical_converter/awr  SystemSampleTime=-1
  awr1_4B : Outport
  wires:
  Emot4_Selection/1 -> awr1/Enable
  Emot1_Selection/1 -> awr/Enable
  nGbxEMIn/1 -> [nGbxEMIn], awr/10
  vltZkBmsPhy/1 -> [vltZkBmsPhy], awr/6
  EMD1_CMD_MotorControlMode/1 -> awr/2
  EMD4_CMD_MotorControlMode/1 -> awr1/2
  [nGbxEMIn] -> awr1/10
  Gain1/1 -> Bus Creator3/1  "EMD4_ACT_DcLinkVoltage"
  Gain/1 -> Bus Creator5/1  "EMD1_ACT_DcLinkVoltage"
  EMD1_CMD_SpeedRefLim/1 -> awr/3
  EMD1_CMD_TorqueRefLim/1 -> awr/4
  HVFreigabeHW_SiRelay_D/1 -> awr/5
  HVFreigabeHW4_SiRelay_D/1 -> awr1/5
  EMD4_CMD_SpeedRefLim/1 -> awr1/3
  EMD4_CMD_Commamd/1 -> awr1/1
  EMD4_CMD_TorqueRefLim/1 -> awr1/4
  Bus Creator4/1 -> awr1_4B/1  "awr1_4B"
  trqEmot4Phy/1 -> awr1/7
  pwEmot4Phy/1 -> awr1/8
  trqEmot4Max/1 -> awr1/9
  trqEmot1Phy/1 -> awr/7
  pwEmot1Phy/1 -> awr/8
  trqEmot1Max/1 -> awr/9
  Bus Creator3/1 -> Switch1/1  "awr4B"
  ZeroWhenNotReady2/1(Out1) -> Switch1/3
  Switch1/1 -> Bus Creator4/2  "awr4B"
  awr1/2 -> Bus Creator3/2
  awr1/3 -> Bus Creator3/3
  awr1/10 -> Bus Creator3/10
  awr1/11 -> Bus Creator3/11
  awr1/5 -> Bus Creator3/5
  awr1/9 -> Bus Creator3/9
  awr1/8 -> Bus Creator3/8
  awr1/7 -> Bus Creator3/7
  awr1/6 -> Bus Creator3/6
  awr1/1 -> Gain1/1
  awr1/4 -> Bus Creator3/4
  ZeroWhenNotReady1/1(Out1) -> Switch2/3
  Switch2/1 -> Bus Creator4/1  "awr1B"
  awr1/12 -> Switch1/2
  awr/9 -> Bus Creator5/9
  awr/7 -> Bus Creator5/7
  awr/6 -> Bus Creator5/6
  awr/10 -> Bus Creator5/10
  awr/11 -> Bus Creator5/11
  awr/8 -> Bus Creator5/8
  awr/5 -> Bus Creator5/5
  awr/4 -> Bus Creator5/4
  awr/1 -> Gain/1
  awr/3 -> Bus Creator5/3
  awr/2 -> Bus Creator5/2
  awr/12 -> Switch2/2
  Bus Creator5/1 -> Switch2/1
  EMD1_CMD_Commamd/1 -> awr/1
  [vltZkBmsPhy] -> awr1/6
  EDCU_Dig_SafetyCutOffDG1/1 -> [EDCU_Dig_SafetyCutOffDG1], awr/11
  [EDCU_Dig_SafetyCutOffDG1] -> awr1/11

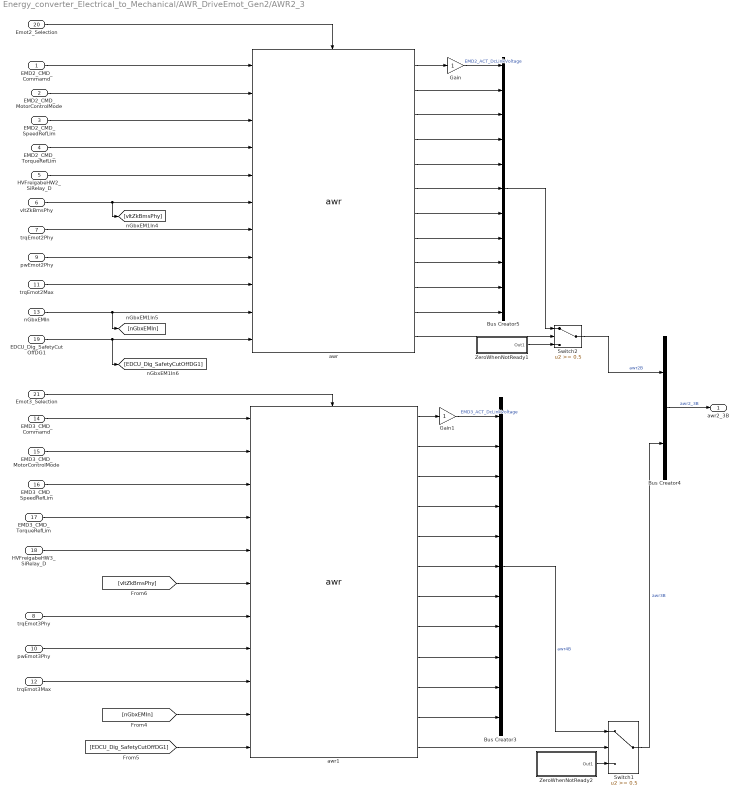
== system Energy_converter_Electrical_to_Mechanical/AWR_DriveEmot_Gen2/AWR2_3 ==
  EMD2_CMD_Commamd : Inport
  EMD2_CMD_MotorControlMode : Inport  Port=2
  EMD2_CMD_SpeedRefLim : Inport  Port=3
  EMD2_CMD_TorqueRefLim : Inport  Port=4
  HVFreigabeHW2_SiRelay_D : Inport  Port=5
  vltZkBmsPhy : Inport  Port=6
  trqEmot2Phy : Inport  Port=7
  trqEmot3Phy : Inport  Port=8
  pwEmot2Phy : Inport  Port=9
  pwEmot3Phy : Inport  Port=10
  trqEmot2Max : Inport  Port=11
  trqEmot3Max : Inport  Port=12
  nGbxEMIn : Inport  Port=13
  EMD3_CMD_Commamd : Inport  Port=14
  EMD3_CMD_MotorControlMode : Inport  Port=15
  EMD3_CMD_SpeedRefLim : Inport  Port=16
  EMD3_CMD_TorqueRefLim : Inport  Port=17
  HVFreigabeHW3_SiRelay_D : Inport  Port=18
  EDCU_Dig_SafetyCutOffDG1 : Inport  Port=19
  Emot2_Selection : Inport  Port=20
  Emot3_Selection : Inport  Port=21
  Bus Creator3 : BusCreator  Inputs=11
  Bus Creator4 : BusCreator  Inputs=2
  Bus Creator5 : BusCreator  Inputs=11
  Gain : Gain
  Gain1 : Gain
  Switch1 : Switch  Threshold=0.5
  Switch2 : Switch  Threshold=0.5
  ZeroWhenNotReady1 : Subsystem  TreatAsAtomicUnit=on
  ZeroWhenNotReady2 : Subsystem  TreatAsAtomicUnit=on
  awr : Electrical_converter/awr  SystemSampleTime=-1
  awr1 : Electrical_converter/awr  SystemSampleTime=-1
  awr2_3B : Outport
  wires:
  Emot3_Selection/1 -> awr1/Enable
  Emot2_Selection/1 -> awr/Enable
  [vltZkBmsPhy] -> awr1/6
  EMD2_CMD_Commamd/1 -> awr/1
  Bus Creator5/1 -> Switch2/1
  awr/12 -> Switch2/2
  awr/2 -> Bus Creator5/2
  awr/3 -> Bus Creator5/3
  awr/1 -> Gain/1
  awr/4 -> Bus Creator5/4
  awr/5 -> Bus Creator5/5
  awr/8 -> Bus Creator5/8
  awr/11 -> Bus Creator5/11
  awr/10 -> Bus Creator5/10
  awr/6 -> Bus Creator5/6
  awr/7 -> Bus Creator5/7
  awr/9 -> Bus Creator5/9
  awr1/12 -> Switch1/2
  Switch2/1 -> Bus Creator4/1  "awr2B"
  ZeroWhenNotReady1/1(Out1) -> Switch2/3
  awr1/4 -> Bus Creator3/4
  awr1/1 -> Gain1/1
  awr1/6 -> Bus Creator3/6
  awr1/7 -> Bus Creator3/7
  awr1/8 -> Bus Creator3/8
  awr1/9 -> Bus Creator3/9
  awr1/5 -> Bus Creator3/5
  awr1/11 -> Bus Creator3/11
  awr1/10 -> Bus Creator3/10
  awr1/3 -> Bus Creator3/3
  awr1/2 -> Bus Creator3/2
  Switch1/1 -> Bus Creator4/2  "awr3B"
  ZeroWhenNotReady2/1(Out1) -> Switch1/3
  Bus Creator3/1 -> Switch1/1  "awr4B"
  trqEmot2Max/1 -> awr/9
  pwEmot2Phy/1 -> awr/8
  trqEmot2Phy/1 -> awr/7
  trqEmot3Max/1 -> awr1/9
  pwEmot3Phy/1 -> awr1/8
  trqEmot3Phy/1 -> awr1/7
  Bus Creator4/1 -> awr2_3B/1  "awr2_3B"
  EMD3_CMD_TorqueRefLim/1 -> awr1/4
  EMD3_CMD_Commamd/1 -> awr1/1
  EMD3_CMD_SpeedRefLim/1 -> awr1/3
  HVFreigabeHW3_SiRelay_D/1 -> awr1/5
  HVFreigabeHW2_SiRelay_D/1 -> awr/5
  EMD2_CMD_TorqueRefLim/1 -> awr/4
  EMD2_CMD_SpeedRefLim/1 -> awr/3
  Gain/1 -> Bus Creator5/1  "EMD2_ACT_DcLinkVoltage"
  Gain1/1 -> Bus Creator3/1  "EMD3_ACT_DcLinkVoltage"
  [nGbxEMIn] -> awr1/10
  EMD3_CMD_MotorControlMode/1 -> awr1/2
  EMD2_CMD_MotorControlMode/1 -> awr/2
  vltZkBmsPhy/1 -> awr/6, [vltZkBmsPhy]
  nGbxEMIn/1 -> awr/10, [nGbxEMIn]
  EDCU_Dig_SafetyCutOffDG1/1 -> [EDCU_Dig_SafetyCutOffDG1], awr/11
  [EDCU_Dig_SafetyCutOffDG1] -> awr1/11

== system Energy_converter_Electrical_to_Mechanical/AWR_DriveEmot_Gen2/EMD1_CMD_Command ==
  EMD1_CMD_ClearErrors : Inport
  EMD1_CMD_MotorControlMode : Inport  Port=2
  Compare To Constant : Subsystem  mask(Compare To Constant){relop===, const=1, OutDataTypeStr=boolean, ZeroCross=on}
      mask prompts: relop "Simulink:masks:Operator_MP"; const "Simulink:masks:ConstantValue_MP"; OutDataTypeStr "Simulink:masks:OutputDataType_MP"; ZeroCross "Simulink:masks:EnableZerocrossingDetection_MP"
      mask help: Simulink:masks:CompareToConstant_MD
      mask init: same as Energy_converter_Electrical_to_Mechanical/AWR_DriveEmot/EMD1_CMD_Command/Compare To Constant
      mask TypeOptions relop: == | ~= | < | <= | >= | >
      mask TypeOptions OutDataTypeStr: Simulink:masks:uint8 | Simulink:masks:boolean
      mask Callback ZeroCross: sl('zeroCrossEnable', gcbh);
      mask Display: disp(str)
  Compare To Constant1 : Subsystem  mask(Compare To Constant){relop===, const=1, OutDataTypeStr=boolean, ZeroCross=on}
      mask prompts: relop "Simulink:masks:Operator_MP"; const "Simulink:masks:ConstantValue_MP"; OutDataTypeStr "Simulink:masks:OutputDataType_MP"; ZeroCross "Simulink:masks:EnableZerocrossingDetection_MP"
      mask help: Simulink:masks:CompareToConstant_MD
      mask init: same as Energy_converter_Electrical_to_Mechanical/AWR_DriveEmot/EMD1_CMD_Command/Compare To Constant
      mask TypeOptions relop: == | ~= | < | <= | >= | >
      mask TypeOptions OutDataTypeStr: Simulink:masks:uint8 | Simulink:masks:boolean
      mask Callback ZeroCross: sl('zeroCrossEnable', gcbh);
      mask Display: disp(str)
  Constant : Constant  Value=4
  Constant3 : Constant
  Constant4 : Constant  Value=0
  Switch : Switch  Threshold=0.5
  Switch1 : Switch  Threshold=0.5
  Out_EMD1_CMD_Command : Outport
  wires:
  Compare To Constant/1(y) -> Switch1/2
  Switch/1 -> Out_EMD1_CMD_Command/1
  Constant4/1 -> Switch1/3
  Constant3/1 -> Switch1/1
  Constant/1 -> Switch/1
  Switch1/1 -> Switch/3
  Compare To Constant1/1(y) -> Switch/2
  EMD1_CMD_ClearErrors/1 -> Compare To Constant1/1(u)
  EMD1_CMD_MotorControlMode/1 -> Compare To Constant/1(u)

== system Energy_converter_Electrical_to_Mechanical/AWR_DriveEmot_Gen2/EMD1_CMD_Command1 ==
  EMD1_CMD_ClearErrors : Inport
  EMD1_CMD_MotorControlMode : Inport  Port=2
  Compare To Constant : Subsystem  mask(Compare To Constant){relop===, const=1, OutDataTypeStr=boolean, ZeroCross=on}
      mask prompts: relop "Simulink:masks:Operator_MP"; const "Simulink:masks:ConstantValue_MP"; OutDataTypeStr "Simulink:masks:OutputDataType_MP"; ZeroCross "Simulink:masks:EnableZerocrossingDetection_MP"
      mask help: Simulink:masks:CompareToConstant_MD
      mask init: same as Energy_converter_Electrical_to_Mechanical/AWR_DriveEmot/EMD1_CMD_Command/Compare To Constant
      mask TypeOptions relop: == | ~= | < | <= | >= | >
      mask TypeOptions OutDataTypeStr: Simulink:masks:uint8 | Simulink:masks:boolean
      mask Callback ZeroCross: sl('zeroCrossEnable', gcbh);
      mask Display: disp(str)
  Compare To Constant1 : Subsystem  mask(Compare To Constant){relop===, const=1, OutDataTypeStr=boolean, ZeroCross=on}
      mask prompts: relop "Simulink:masks:Operator_MP"; const "Simulink:masks:ConstantValue_MP"; OutDataTypeStr "Simulink:masks:OutputDataType_MP"; ZeroCross "Simulink:masks:EnableZerocrossingDetection_MP"
      mask help: Simulink:masks:CompareToConstant_MD
      mask init: same as Energy_converter_Electrical_to_Mechanical/AWR_DriveEmot/EMD1_CMD_Command/Compare To Constant
      mask TypeOptions relop: == | ~= | < | <= | >= | >
      mask TypeOptions OutDataTypeStr: Simulink:masks:uint8 | Simulink:masks:boolean
      mask Callback ZeroCross: sl('zeroCrossEnable', gcbh);
      mask Display: disp(str)
  Constant : Constant  Value=4
  Constant3 : Constant
  Constant4 : Constant  Value=0
  Switch : Switch  Threshold=0.5
  Switch1 : Switch  Threshold=0.5
  Out_EMD1_CMD_Command : Outport
  wires:
  Compare To Constant/1(y) -> Switch1/2
  Switch/1 -> Out_EMD1_CMD_Command/1
  Constant4/1 -> Switch1/3
  Constant3/1 -> Switch1/1
  Constant/1 -> Switch/1
  Switch1/1 -> Switch/3
  Compare To Constant1/1(y) -> Switch/2
  EMD1_CMD_ClearErrors/1 -> Compare To Constant1/1(u)
  EMD1_CMD_MotorControlMode/1 -> Compare To Constant/1(u)

== system Energy_converter_Electrical_to_Mechanical/AWR_DriveEmot_Gen2/EMD1_CMD_Command2 ==
  EMD1_CMD_ClearErrors : Inport
  EMD1_CMD_MotorControlMode : Inport  Port=2
  Compare To Constant : Subsystem  mask(Compare To Constant){relop===, const=1, OutDataTypeStr=boolean, ZeroCross=on}
      mask prompts: relop "Simulink:masks:Operator_MP"; const "Simulink:masks:ConstantValue_MP"; OutDataTypeStr "Simulink:masks:OutputDataType_MP"; ZeroCross "Simulink:masks:EnableZerocrossingDetection_MP"
      mask help: Simulink:masks:CompareToConstant_MD
      mask init: same as Energy_converter_Electrical_to_Mechanical/AWR_DriveEmot/EMD1_CMD_Command/Compare To Constant
      mask TypeOptions relop: == | ~= | < | <= | >= | >
      mask TypeOptions OutDataTypeStr: Simulink:masks:uint8 | Simulink:masks:boolean
      mask Callback ZeroCross: sl('zeroCrossEnable', gcbh);
      mask Display: disp(str)
  Compare To Constant1 : Subsystem  mask(Compare To Constant){relop===, const=1, OutDataTypeStr=boolean, ZeroCross=on}
      mask prompts: relop "Simulink:masks:Operator_MP"; const "Simulink:masks:ConstantValue_MP"; OutDataTypeStr "Simulink:masks:OutputDataType_MP"; ZeroCross "Simulink:masks:EnableZerocrossingDetection_MP"
      mask help: Simulink:masks:CompareToConstant_MD
      mask init: same as Energy_converter_Electrical_to_Mechanical/AWR_DriveEmot/EMD1_CMD_Command/Compare To Constant
      mask TypeOptions relop: == | ~= | < | <= | >= | >
      mask TypeOptions OutDataTypeStr: Simulink:masks:uint8 | Simulink:masks:boolean
      mask Callback ZeroCross: sl('zeroCrossEnable', gcbh);
      mask Display: disp(str)
  Constant : Constant  Value=4
  Constant3 : Constant
  Constant4 : Constant  Value=0
  Switch : Switch  Threshold=0.5
  Switch1 : Switch  Threshold=0.5
  Out_EMD1_CMD_Command : Outport
  wires:
  Compare To Constant/1(y) -> Switch1/2
  Switch/1 -> Out_EMD1_CMD_Command/1
  Constant4/1 -> Switch1/3
  Constant3/1 -> Switch1/1
  Constant/1 -> Switch/1
  Switch1/1 -> Switch/3
  Compare To Constant1/1(y) -> Switch/2
  EMD1_CMD_ClearErrors/1 -> Compare To Constant1/1(u)
  EMD1_CMD_MotorControlMode/1 -> Compare To Constant/1(u)

== system Energy_converter_Electrical_to_Mechanical/AWR_DriveEmot_Gen2/EMD1_CMD_Command3 ==
  EMD1_CMD_ClearErrors : Inport
  EMD1_CMD_MotorControlMode : Inport  Port=2
  Compare To Constant : Subsystem  mask(Compare To Constant){relop===, const=1, OutDataTypeStr=boolean, ZeroCross=on}
      mask prompts: relop "Simulink:masks:Operator_MP"; const "Simulink:masks:ConstantValue_MP"; OutDataTypeStr "Simulink:masks:OutputDataType_MP"; ZeroCross "Simulink:masks:EnableZerocrossingDetection_MP"
      mask help: Simulink:masks:CompareToConstant_MD
      mask init: same as Energy_converter_Electrical_to_Mechanical/AWR_DriveEmot/EMD1_CMD_Command/Compare To Constant
      mask TypeOptions relop: == | ~= | < | <= | >= | >
      mask TypeOptions OutDataTypeStr: Simulink:masks:uint8 | Simulink:masks:boolean
      mask Callback ZeroCross: sl('zeroCrossEnable', gcbh);
      mask Display: disp(str)
  Compare To Constant1 : Subsystem  mask(Compare To Constant){relop===, const=1, OutDataTypeStr=boolean, ZeroCross=on}
      mask prompts: relop "Simulink:masks:Operator_MP"; const "Simulink:masks:ConstantValue_MP"; OutDataTypeStr "Simulink:masks:OutputDataType_MP"; ZeroCross "Simulink:masks:EnableZerocrossingDetection_MP"
      mask help: Simulink:masks:CompareToConstant_MD
      mask init: same as Energy_converter_Electrical_to_Mechanical/AWR_DriveEmot/EMD1_CMD_Command/Compare To Constant
      mask TypeOptions relop: == | ~= | < | <= | >= | >
      mask TypeOptions OutDataTypeStr: Simulink:masks:uint8 | Simulink:masks:boolean
      mask Callback ZeroCross: sl('zeroCrossEnable', gcbh);
      mask Display: disp(str)
  Constant : Constant  Value=4
  Constant3 : Constant
  Constant4 : Constant  Value=0
  Switch : Switch  Threshold=0.5
  Switch1 : Switch  Threshold=0.5
  Out_EMD1_CMD_Command : Outport
  wires:
  Compare To Constant/1(y) -> Switch1/2
  Switch/1 -> Out_EMD1_CMD_Command/1
  Constant4/1 -> Switch1/3
  Constant3/1 -> Switch1/1
  Constant/1 -> Switch/1
  Switch1/1 -> Switch/3
  Compare To Constant1/1(y) -> Switch/2
  EMD1_CMD_ClearErrors/1 -> Compare To Constant1/1(u)
  EMD1_CMD_MotorControlMode/1 -> Compare To Constant/1(u)

== system Energy_converter_Electrical_to_Mechanical/AWR_DriveEmot_Gen2/Emot1_4 ==
  nGbxEMIn : Inport
  voltBatHV1 : Inport  Port=2
  trqEmotDesPhy1 : Inport  Port=3
  emot_CMD1 : Inport  Port=4
  emot_oil_temperature1 : Inport  Port=5
  inv_coolant_temperature1 : Inport  Port=6
  voltBatHV4 : Inport  Port=7
  trqEmotDesPhy4 : Inport  Port=8
  emot_CMD4 : Inport  Port=9
  emot_oil_temperature4 : Inport  Port=10
  inv_coolant_temperature4 : Inport  Port=11
  Emot1_Selection : Inport  Port=12
  Emot4_Selection : Inport  Port=13
  Bus Creator1 : BusCreator  Inputs=9
  Bus Creator2 : BusCreator  Inputs=9
  Bus Creator3 : BusCreator  Inputs=2
  e-Motor_Gen2 : Energy_converter_Electrical_to_Mechanical/e-Motor_Gen2  SystemSampleTime=-1
  e-Motor_Gen2_1 : Energy_converter_Electrical_to_Mechanical/e-Motor_Gen2  SystemSampleTime=-1
  emot1_4B : Outport
  wires:
  Emot4_Selection/1 -> e-Motor_Gen2_1/Enable
  Emot1_Selection/1 -> e-Motor_Gen2/Enable
  emot_CMD1/1 -> e-Motor_Gen2/4
  e-Motor_Gen2/5 -> Bus Creator1/5
  e-Motor_Gen2/2 -> Bus Creator1/2
  e-Motor_Gen2/1 -> Bus Creator1/1
  e-Motor_Gen2/4 -> Bus Creator1/4
  e-Motor_Gen2/3 -> Bus Creator1/3
  nGbxEMIn/1 -> [nGbxEMIn], e-Motor_Gen2/1
  trqEmotDesPhy1/1 -> e-Motor_Gen2/3
  voltBatHV1/1 -> e-Motor_Gen2/2
  Bus Creator1/1 -> Bus Creator3/1  "emot1B"
  Bus Creator3/1 -> emot1_4B/1  "emot1_4B"
  e-Motor_Gen2/6 -> Bus Creator1/6
  e-Motor_Gen2/7 -> Bus Creator1/7
  e-Motor_Gen2/8 -> Bus Creator1/8
  e-Motor_Gen2/9 -> Bus Creator1/9
  Bus Creator2/1 -> Bus Creator3/2  "emot4B"
  e-Motor_Gen2_1/1 -> Bus Creator2/1
  e-Motor_Gen2_1/2 -> Bus Creator2/2
  e-Motor_Gen2_1/3 -> Bus Creator2/3
  e-Motor_Gen2_1/4 -> Bus Creator2/4
  e-Motor_Gen2_1/5 -> Bus Creator2/5
  e-Motor_Gen2_1/6 -> Bus Creator2/6
  e-Motor_Gen2_1/7 -> Bus Creator2/7
  e-Motor_Gen2_1/8 -> Bus Creator2/8
  e-Motor_Gen2_1/9 -> Bus Creator2/9
  [nGbxEMIn] -> e-Motor_Gen2_1/1
  voltBatHV4/1 -> e-Motor_Gen2_1/2
  trqEmotDesPhy4/1 -> e-Motor_Gen2_1/3
  emot_CMD4/1 -> e-Motor_Gen2_1/4
  emot_oil_temperature1/1 -> e-Motor_Gen2/5
  inv_coolant_temperature1/1 -> e-Motor_Gen2/6
  emot_oil_temperature4/1 -> e-Motor_Gen2_1/5
  inv_coolant_temperature4/1 -> e-Motor_Gen2_1/6

== system Energy_converter_Electrical_to_Mechanical/AWR_DriveEmot_Gen2/Emot2_3 ==
  nGbxEMIn : Inport
  voltBatHV2 : Inport  Port=2
  trqEmotDesPhy2 : Inport  Port=3
  emot_CMD2 : Inport  Port=4
  emot_oil_temperature2 : Inport  Port=5
  inv_coolant_temperature2 : Inport  Port=6
  voltBatHV3 : Inport  Port=7
  trqEmotDesPhy3 : Inport  Port=8
  emot_CMD3 : Inport  Port=9
  emot_oil_temperature3 : Inport  Port=10
  inv_coolant_temperature3 : Inport  Port=11
  Emot2_Selection : Inport  Port=12
  Emot3_Selection : Inport  Port=13
  Bus Creator1 : BusCreator  Inputs=9
  Bus Creator2 : BusCreator  Inputs=9
  Bus Creator3 : BusCreator  Inputs=2
  e-Motor_Gen2 : Energy_converter_Electrical_to_Mechanical/e-Motor_Gen2  SystemSampleTime=-1
  e-Motor_Gen2_1 : Energy_converter_Electrical_to_Mechanical/e-Motor_Gen2  SystemSampleTime=-1
  emot2_3B : Outport
  wires:
  Emot3_Selection/1 -> e-Motor_Gen2_1/Enable
  Emot2_Selection/1 -> e-Motor_Gen2/Enable
  Bus Creator3/1 -> emot2_3B/1  "emot2_3B"
  trqEmotDesPhy3/1 -> e-Motor_Gen2_1/3
  Bus Creator2/1 -> Bus Creator3/2  "emot3B"
  Bus Creator1/1 -> Bus Creator3/1  "emot2B"
  voltBatHV3/1 -> e-Motor_Gen2_1/2
  [nGbxEMIn] -> e-Motor_Gen2_1/1
  voltBatHV2/1 -> e-Motor_Gen2/2
  trqEmotDesPhy2/1 -> e-Motor_Gen2/3
  nGbxEMIn/1 -> [nGbxEMIn], e-Motor_Gen2/1
  e-Motor_Gen2/3 -> Bus Creator1/3
  e-Motor_Gen2/4 -> Bus Creator1/4
  e-Motor_Gen2/1 -> Bus Creator1/1
  e-Motor_Gen2/2 -> Bus Creator1/2
  e-Motor_Gen2/5 -> Bus Creator1/5
  e-Motor_Gen2_1/1 -> Bus Creator2/1
  e-Motor_Gen2_1/2 -> Bus Creator2/2
  e-Motor_Gen2_1/3 -> Bus Creator2/3
  e-Motor_Gen2_1/4 -> Bus Creator2/4
  e-Motor_Gen2_1/5 -> Bus Creator2/5
  emot_CMD2/1 -> e-Motor_Gen2/4
  emot_CMD3/1 -> e-Motor_Gen2_1/4
  e-Motor_Gen2/6 -> Bus Creator1/6
  e-Motor_Gen2/7 -> Bus Creator1/7
  e-Motor_Gen2/8 -> Bus Creator1/8
  e-Motor_Gen2/9 -> Bus Creator1/9
  e-Motor_Gen2_1/6 -> Bus Creator2/6
  e-Motor_Gen2_1/7 -> Bus Creator2/7
  e-Motor_Gen2_1/8 -> Bus Creator2/8
  e-Motor_Gen2_1/9 -> Bus Creator2/9
  emot_oil_temperature2/1 -> e-Motor_Gen2/5
  inv_coolant_temperature2/1 -> e-Motor_Gen2/6
  inv_coolant_temperature3/1 -> e-Motor_Gen2_1/6
  emot_oil_temperature3/1 -> e-Motor_Gen2_1/5

== system Energy_converter_Electrical_to_Mechanical/AWR_DriveEmot_Gen2/MotorSelection ==
  MidAxle : Constant  Value=midAxleNoOfEmot
  RearAxle : Constant  Value=rearAxleNoOfEmot
  Truth Table : Truth Table  TreatAsAtomicUnit=on
  Emot1_Selection : Outport
  Emot2_Selection : Outport  Port=2
  Emot3_Selection : Outport  Port=3
  Emot4_Selection : Outport  Port=4
  wires:
  Truth Table/4(y4) -> Emot4_Selection/1
  Truth Table/3(y3) -> Emot3_Selection/1
  Truth Table/2(y2) -> Emot2_Selection/1
  Truth Table/1(y1) -> Emot1_Selection/1
  RearAxle/1 -> Truth Table/2(u2)
  MidAxle/1 -> Truth Table/1(u1)
